simulink model "slb_scalar_vector"  (R2015b)
settings: Solver=FixedStepDiscrete  SolverMode=SingleTasking  StartTime=0.0  StopTime=3  RelTol=1e-3
settings Model: Creator=at-mt  LastModifiedBy=amatsumo
settings DataIOCC: SaveFormat=Array  SignalLoggingSaveFormat=ModelDataLogs  SaveOutput=off  SignalLogging=off  SaveTime=off
settings OptimizationCC: BlockReduction=off  ConditionallyExecuteInputs=off  DefaultParameterBehavior=Inlined  ExpressionDepthLimit=2147483647
settings DebuggingCC: AlgebraicLoopMsg=error  UnderspecifiedInitializationDetection=Classic  MergeDetectMultiDrivingBlocksExec=none  SolverPrmCheckMsg=warning  SingleTaskRateTransMsg=error  FcnCallInpInsideContextMsg=UseLocalSettings  StateNameClashWarn=warning
settings HardwareCC: ProdBitPerPointer=32  ProdLargestAtomicFloat=None  ProdIntDivRoundTo=Undefined  ProdEndianess=Unspecified  ProdWordSize=32  ProdHWDeviceType=ASIC/FPGA->ASIC/FPGA  ProdEqTarget=off
settings SFSimCC: SFSimEcho=off
settings GRTTargetCC: GeneratePreprocessorConditionals=Disable all  CombineOutputUpdateFcns=off  GRTInterface=on
settings ConfigComp: CovModelRefEnable=Off  CovSFcnEnable=off

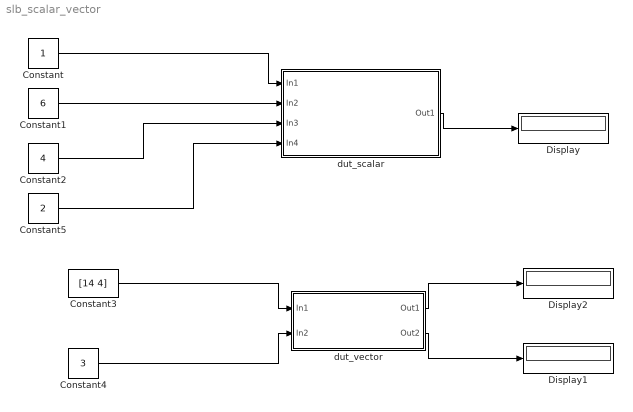
== system slb_scalar_vector ==
  Constant : Constant  OutDataTypeStr=int8  SampleTime=1
  Constant1 : Constant  Value=6  OutDataTypeStr=int8  SampleTime=1
  Constant2 : Constant  Value=4  OutDataTypeStr=int8  SampleTime=1
  Constant3 : Constant  Value=[14 4]  OutDataTypeStr=int8  SampleTime=1
  Constant4 : Constant  Value=3  OutDataTypeStr=int8  SampleTime=1
  Constant5 : Constant  Value=2  OutDataTypeStr=int8  SampleTime=1
  Display : Display
  Display1 : Display
  Display2 : Display
  dut_scalar : Subsystem
  dut_vector : Subsystem
  wires:
  Constant/1 -> dut_scalar/1(In1)
  Constant1/1 -> dut_scalar/2(In2)
  dut_scalar/1(Out1) -> Display/1
  Constant3/1 -> dut_vector/1(In1)
  Constant4/1 -> dut_vector/2(In2)
  dut_vector/2(Out2) -> Display1/1
  dut_vector/1(Out1) -> Display2/1
  Constant2/1 -> dut_scalar/3(In3)
  Constant5/1 -> dut_scalar/4(In4)

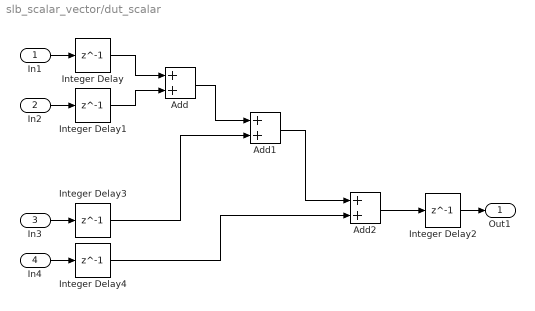
== system slb_scalar_vector/dut_scalar ==
  In1 : Inport
  In2 : Inport  Port=2
  In3 : Inport  Port=3
  In4 : Inport  Port=4
  Add : Sum  OutDataTypeStr=fixdt(1,7,0)  RndMeth=Nearest
  Add1 : Sum  RndMeth=Nearest  OutDataTypeStr=Inherit: Same as first input
  Add2 : Sum  RndMeth=Nearest  OutDataTypeStr=Inherit: Same as first input
  Integer Delay{,1..4} (5 alike) : Delay  DelayLength=1  InputProcessing=Inherited
  Out1 : Outport
  wires:
  Integer Delay/1 -> Add/1
  Integer Delay1/1 -> Add/2
  Add/1 -> Add1/1
  Integer Delay3/1 -> Add1/2
  In1/1 -> Integer Delay/1
  In2/1 -> Integer Delay1/1
  Integer Delay2/1 -> Out1/1
  In3/1 -> Integer Delay3/1
  In4/1 -> Integer Delay4/1
  Add1/1 -> Add2/1
  Integer Delay4/1 -> Add2/2
  Add2/1 -> Integer Delay2/1

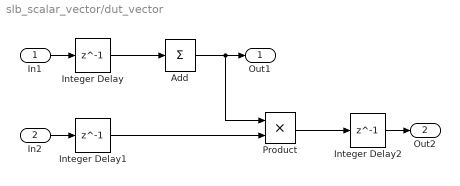
== system slb_scalar_vector/dut_vector ==
  In1 : Inport
  In2 : Inport  Port=2
  Add : Sum  Inputs=+
  Integer Delay : Delay  DelayLength=1  InputProcessing=Inherited
  Integer Delay1 : Delay  DelayLength=1  InputProcessing=Inherited
  Integer Delay2 : Delay  DelayLength=1  InputProcessing=Inherited
  Product : Product  RndMeth=Zero
  Out1 : Outport
  Out2 : Outport  Port=2
  wires:
  In2/1 -> Integer Delay1/1
  Integer Delay2/1 -> Out2/1
  In1/1 -> Integer Delay/1
  Integer Delay1/1 -> Product/2
  Product/1 -> Integer Delay2/1
  Add/1 -> Out1/1, Product/1
  Integer Delay/1 -> Add/1
